simulink library "speedgoatlib"  (Simulink 7.5)
settings: Solver=ode45  StartTime=0.0  StopTime=10.0  RelTol=1e-3
undefined symbols (not defined in the file): m_XR17D15x, mmodemcontrol, standard
libraries: speedgoatlib x176, xpclib x88, simulink x4
(part 2 of 4)

== system speedgoatlib/IO503 ==
  Send Receive : Subsystem  InitFcn=m_XR17D15x(3);  mask(sendreceive_IO503){group=Basic Setup, port=1, irqnum=5, slot=-1, transceiver1=RS232 (max 921.6kb/s), standard1=on, baud1=115200, bauddivisor1=1, sampling1=16x (standard), prescale1=off, parity1=None, ndata1=8, nstop1=1, rlevel1=1, hwmode1=none, swmode1=none, xonchar1=17, xoffchar1=19, rs485auto1=off, rs485delay1=0, xmtfifosize1=1024, xmtdatatype1=8 bit uint null terminated, rcvfifosize1=1024, transceiver2=RS232 (max 921.6kb/s), standard2=on, baud2=115200, bauddivisor2=1, sampling2=16x (standard), prescale2=off, parity2=None, ndata2=8, nstop2=1, rlevel2=1, hwmode2=none, swmode2=none, xonchar2=17, xoffchar2=19, rs485auto2=off, rs485delay2=0, xmtfifosize2=1024, xmtdatatype2=8 bit uint null terminated, rcvfifosize2=1024, transceiver3=RS232 (max 921.6kb/s), standard3=on, baud3=115200, bauddivisor3=1, sampling3=16x (standard), prescale3=off, parity3=None, ndata3=8, nstop3=1, rlevel3=half full (32), hwmode3=none, swmode3=none, xonchar3=17, xoffchar3=19, rs485auto3=off, rs485delay3=0, xmtfifosize3=1024, xmtdatatype3=8 bit uint null terminated, rcvfifosize3=1024, transceiver4=RS232 (max 921.6kb/s), standard4=on, baud4=115200, bauddivisor4=1, sampling4=16x (standard), prescale4=off, parity4=None, ndata4=8, nstop4=1, rlevel4=half full (32), hwmode4=none, swmode4=none, xonchar4=17, xoffchar4=19, rs485auto4=off, rs485delay4=0, xmtfifosize4=1024, xmtdatatype4=8 bit uint null terminated, rcvfifosize4=1024}
      mask prompts: group "Parameter group:"; port "Port to modify:"; irqnum "IRQ number:"; slot "PCI slot (-1: autosearch):"; transceiver1 "Transceiver setup:"; standard1 "Use standard baud rates (16x, no prescaling)"; baud1 "Standard baud rate:"; bauddivisor1 "Baud rate divisor (non-standard baud rates):"; sampling1 "Sampling rate (non-standard baud rates):"; prescale1 "Prescale by 4 (non-standard baud rates)"; parity1 "Parity:"; ndata1 "Data bits:"; nstop1 "Stop bits:"; rlevel1 "Receive FIFO interrupt level:"; hwmode1 "Hardware handshake:"; swmode1 "Software handshake:"; xonchar1 "XON character:"; xoffchar1 "XOFF character:"; rs485auto1 "RS485 auto turnaround:"; rs485delay1 "RS485 turnaround delay [0,15]"; xmtfifosize1 "Transmit software FIFO size:"; xmtdatatype1 "Transmit FIFO data type:"; rcvfifosize1 "Receive software FIFO size:"; transceiver2 "Transceiver setup:"; standard2 "Use standard baud rates (16x, no prescaling)"; baud2 "Standard baud rate:"; bauddivisor2 "Baud rate divisor (non-standard baud rates):"; sampling2 "Sampling rate (non-standard baud rates):"; prescale2 "Prescale by 4 (non-standard baud rates)"; parity2 "Parity:"; ndata2 "Data bits:"; nstop2 "Stop bits:"; rlevel2 "Receive FIFO interrupt level:"; hwmode2 "Hardware handshake:"; swmode2 "Software handshake:"; xonchar2 "XON character:"; xoffchar2 "XOFF character:"; rs485auto2 "RS485 auto turnaround:"; rs485delay2 "RS485 turnaround delay [0,15]"; xmtfifosize2 "Transmit software FIFO size:"; xmtdatatype2 "Transmit FIFO data type:"; rcvfifosize2 "Receive software FIFO size:"; transceiver3 "Transceiver setup:"; standard3 "Use standard baud rates (16x, no prescaling)"; baud3 "Standard baud rate:"; bauddivisor3 "Baud rate divisor (non-standard baud rates):"; sampling3 "Sampling rate (non-standard baud rates):"; prescale3 "Prescale by 4 (non-standard baud rates)"; parity3 "Parity:"; ndata3 "Data bits:"; nstop3 "Stop bits:"; rlevel3 "Receive FIFO interrupt level:"; hwmode3 "Hardware handshake:"; swmode3 "Software handshake:"; xonchar3 "XON character:"; xoffchar3 "XOFF character:"; rs485auto3 "RS485 auto turnaround:"; rs485delay3 "RS485 turnaround delay [0,15]"; xmtfifosize3 "Transmit software FIFO size:"; xmtdatatype3 "Transmit FIFO data type:"; rcvfifosize3 "Receive software FIFO size:"; transceiver4 "Transceiver setup:"; standard4 "Use standard baud rates (16x, no prescaling)"; baud4 "Standard baud rate:"; bauddivisor4 "Baud rate divisor (non-standard baud rates):"; sampling4 "Sampling rate (non-standard baud rates):"; prescale4 "Prescale by 4 (non-standard baud rates)"; parity4 "Parity:"; ndata4 "Data bits:"; nstop4 "Stop bits:"; rlevel4 "Receive FIFO interrupt level:"; hwmode4 "Hardware handshake:"; swmode4 "Software handshake:"; xonchar4 "XON character:"; xoffchar4 "XOFF character:"; rs485auto4 "RS485 auto turnaround:"; rs485delay4 "RS485 turnaround delay [0,15]"; xmtfifosize4 "Transmit software FIFO size:"; xmtdatatype4 "Transmit FIFO data type:"; rcvfifosize4 "Receive software FIFO size:"
      mask help:
      | Speedgoat driver block
      | IO503 - Send Receive
      mask init:
      | brdslot = slot;
      | m_tews_XR17D15x(1, 4);
      mask Help: web(fullfile(speedgoatroot,'sg_help','serial','dialog_fields_send_rec_io503.htm'),'-helpbrowser');
      mask StyleString: popup(Board Setup|Basic Setup|FIFO Setup),popup(1|2|3|4),edit,edit,popup(RS232 (max 921.6kb/s)|RS422|RS422 multidrop|RS485 full-duplex|RS485 half-duplex),checkbox,popup(2764800|1382400|921600|460800|230400|115200|57600|38400|19200|9600|4800|2400|1200|600|400),edit,popup(8x|16x (standard)),checkbox,popup(None|Even|Odd|Mark|Space),popup(5|6|7|8),popup(1|2),popup(1|quarter full (16)|half full (32)|almost full (56)),popup(RTS/CTS|none),popup(XON/XOFF|none),edit,edit,checkbox,edit,edit,popup(count+32 bit int|count+32 bit uint|count+16 bit int|count+16 bit uint|8 bit int null terminated|8 bit uint null terminated),edit,popup(RS232 (max 921.6kb/s)|RS422|RS422 multidrop|RS485 full-duplex|RS485 half-duplex),checkbox,popup(2764800|1382400|921600|460800|230400|115200|57600|38400|19200|9600|4800|2400|1200|600|400),edit,popup(8x|16x (standard)),checkbox,popup(None|Even|Odd|Mark|Space),popup(5|6|7|8),popup(1|2),popup(1|quarter full (16)|half full (32)|almost full (56)),popup(RTS/CTS|none),popup(XON/XOFF|none),edit,edit,checkbox,edit,edit,popup(count+32 bit int|count+32 bit uint|count+16 bit int|count+16 bit uint|8 bit int null terminated|8 bit uint null terminated),edit,popup(RS232 (max 921.6kb/s)|RS422|RS422 multidrop|RS485 full-duplex|RS485 half-duplex),checkbox,popup(2764800|1382400|921600|460800|230400|115200|57600|38400|19200|9600|4800|2400|1200|600|400),edit,popup(8x|16x (standard)),checkbox,popup(None|Even|Odd|Mark|Space),popup(5|6|7|8),popup(1|2),popup(1|quarter full (16)|half full (32)|almost full (56)),popup(RTS/CTS|none),popup(XON/XOFF|none),edit,edit,checkbox,edit,edit,popup(count+32 bit int|count+32 bit uint|count+16 bit int|count+16 bit uint|8 bit int null terminated|8 bit uint null terminated),edit,popup(RS232 (max 921.6kb/s)|RS422|RS422 multidrop|RS485 full-duplex|RS485 half-duplex),checkbox,popup(2764800|1382400|921600|460800|230400|115200|57600|38400|19200|9600|4800|2400|1200|600|400),edit,popup(8x|16x (standard)),checkbox,popup(None|Even|Odd|Mark|Space),popup(5|6|7|8),popup(1|2),popup(1|quarter full (16)|half full (32)|almost full (56)),popup(RTS/CTS|none),popup(XON/XOFF|none),edit,edit,checkbox,edit,edit,popup(count+32 bit int|count+32 bit uint|count+16 bit int|count+16 bit uint|8 bit int null terminated|8 bit uint null terminated),edit
      mask CallbackString: m_tews_XR17D15x(2, 4);|m_tews_XR17D15x(2, 4);||||||||||||||||||||||||||||||||||||||||||||||||||||||||||||||||||||||||||||||
      mask Display:
      | disp('Speedgoat\nIO503\nRS232/422/485\nSend\nReceive');
      | port_label( 'input', 1, 'XMT1' );
      | port_label( 'input', 2, 'XMT2' );
      | port_label( 'input', 3, 'XMT3' );
      | port_label( 'input', 4, 'XMT4' );
      | 
      | port_label( 'output', 1, 'FIFO1' );
      | port_label( 'output', 2, 'FIFO2' );
      | port_label( 'output', 3, 'FIFO3' );
      | port_label( 'output', 4, 'FIFO4' );
  Speedgoat IO503 Internal blocks : Subsystem

== system speedgoatlib/IO504 ==
  Send Receive : Subsystem  InitFcn=m_XR17D15x(3);  mask(sendreceive_IO504){group=Basic Setup, port=1, irqnum=5, slot=-1, transceiver1=RS232 (max 921.6kb/s), standard1=on, baud1=115200, bauddivisor1=1, sampling1=16x (standard), prescale1=off, parity1=None, ndata1=8, nstop1=1, rlevel1=1, hwmode1=none, swmode1=none, xonchar1=17, xoffchar1=19, rs485auto1=off, rs485delay1=0, xmtfifosize1=1024, xmtdatatype1=8 bit uint null terminated, rcvfifosize1=1024, transceiver2=RS232 (max 921.6kb/s), standard2=on, baud2=115200, bauddivisor2=1, sampling2=16x (standard), prescale2=off, parity2=None, ndata2=8, nstop2=1, rlevel2=1, hwmode2=none, swmode2=none, xonchar2=17, xoffchar2=19, rs485auto2=off, rs485delay2=0, xmtfifosize2=1024, xmtdatatype2=8 bit uint null terminated, rcvfifosize2=1024, transceiver3=RS232 (max 921.6kb/s), standard3=on, baud3=115200, bauddivisor3=1, sampling3=16x (standard), prescale3=off, parity3=None, ndata3=8, nstop3=1, rlevel3=half full (32), hwmode3=none, swmode3=none, xonchar3=17, xoffchar3=19, rs485auto3=off, rs485delay3=0, xmtfifosize3=1024, xmtdatatype3=8 bit uint null terminated, rcvfifosize3=1024, transceiver4=RS232 (max 921.6kb/s), standard4=on, baud4=115200, bauddivisor4=1, sampling4=16x (standard), prescale4=off, parity4=None, ndata4=8, nstop4=1, rlevel4=half full (32), hwmode4=none, swmode4=none, xonchar4=17, xoffchar4=19, rs485auto4=off, rs485delay4=0, xmtfifosize4=1024, xmtdatatype4=8 bit uint null terminated, rcvfifosize4=1024, transceiver5=RS232 (max 921.6kb/s), standard5=on, baud5=115200, bauddivisor5=1, sampling5=16x (standard), prescale5=off, parity5=None, ndata5=8, nstop5=1, rlevel5=1, hwmode5=none, swmode5=none, xonchar5=17, xoffchar5=19, rs485auto5=off, rs485delay5=0, xmtfifosize5=1024, xmtdatatype5=8 bit uint null terminated, rcvfifosize5=1024, transceiver6=RS232 (max 921.6kb/s), standard6=on, baud6=115200, bauddivisor6=1, sampling6=16x (standard), prescale6=off, parity6=None, ndata6=8, nstop6=1, rlevel6=1, hwmode6=none, swmode6=none, xonchar6=17, xoffchar6=19, rs485auto6=off, rs485delay6=0, xmtfifosize6=1024, xmtdatatype6=8 bit uint null terminated, rcvfifosize6=1024, transceiver7=RS232 (max 921.6kb/s), standard7=on, baud7=115200, bauddivisor7=1, sampling7=16x (standard), prescale7=off, parity7=None, ndata7=8, nstop7=1, rlevel7=1, hwmode7=none, swmode7=none, xonchar7=17, xoffchar7=19, rs485auto7=off, rs485delay7=0, xmtfifosize7=1024, xmtdatatype7=8 bit uint null terminated, rcvfifosize7=1024, transceiver8=RS232 (max 921.6kb/s), standard8=on, baud8=115200, bauddivisor8=1, sampling8=16x (standard), prescale8=off, parity8=None, ndata8=8, nstop8=1, rlevel8=1, hwmode8=none, swmode8=none, xonchar8=17, xoffchar8=19, rs485auto8=off, rs485delay8=0, xmtfifosize8=1024, xmtdatatype8=8 bit uint null terminated, rcvfifosize8=1024}
      mask prompts: group "Parameter group:"; port "Port to modify:"; irqnum "IRQ number:"; slot "PCI slot (-1: autosearch):"; transceiver1 "Transceiver setup:"; standard1 "Use standard baud rates (16x, no prescaling)"; baud1 "Standard baud rate:"; bauddivisor1 "Baud rate divisor (non-standard baud rates):"; sampling1 "Sampling rate (non-standard baud rates):"; prescale1 "Prescale by 4 (non-standard baud rates)"; parity1 "Parity:"; ndata1 "Data bits:"; nstop1 "Stop bits:"; rlevel1 "Receive FIFO interrupt level:"; hwmode1 "Hardware handshake:"; swmode1 "Software handshake:"; xonchar1 "XON character:"; xoffchar1 "XOFF character:"; rs485auto1 "RS485 auto turnaround:"; rs485delay1 "RS485 turnaround delay [0,15]"; xmtfifosize1 "Transmit software FIFO size:"; xmtdatatype1 "Transmit FIFO data type:"; rcvfifosize1 "Receive software FIFO size:"; transceiver2 "Transceiver setup:"; standard2 "Use standard baud rates (16x, no prescaling)"; baud2 "Standard baud rate:"; bauddivisor2 "Baud rate divisor (non-standard baud rates):"; sampling2 "Sampling rate (non-standard baud rates):"; prescale2 "Prescale by 4 (non-standard baud rates)"; parity2 "Parity:"; ndata2 "Data bits:"; nstop2 "Stop bits:"; rlevel2 "Receive FIFO interrupt level:"; hwmode2 "Hardware handshake:"; swmode2 "Software handshake:"; xonchar2 "XON character:"; xoffchar2 "XOFF character:"; rs485auto2 "RS485 auto turnaround:"; rs485delay2 "RS485 turnaround delay [0,15]"; xmtfifosize2 "Transmit software FIFO size:"; xmtdatatype2 "Transmit FIFO data type:"; rcvfifosize2 "Receive software FIFO size:"; transceiver3 "Transceiver setup:"; standard3 "Use standard baud rates (16x, no prescaling)"; baud3 "Standard baud rate:"; bauddivisor3 "Baud rate divisor (non-standard baud rates):"; sampling3 "Sampling rate (non-standard baud rates):"; prescale3 "Prescale by 4 (non-standard baud rates)"; parity3 "Parity:"; ndata3 "Data bits:"; nstop3 "Stop bits:"; rlevel3 "Receive FIFO interrupt level:"; hwmode3 "Hardware handshake:"; swmode3 "Software handshake:"; xonchar3 "XON character:"; xoffchar3 "XOFF character:"; rs485auto3 "RS485 auto turnaround:"; rs485delay3 "RS485 turnaround delay [0,15]"; xmtfifosize3 "Transmit software FIFO size:"; xmtdatatype3 "Transmit FIFO data type:"; rcvfifosize3 "Receive software FIFO size:"; transceiver4 "Transceiver setup:"; standard4 "Use standard baud rates (16x, no prescaling)"; baud4 "Standard baud rate:"; bauddivisor4 "Baud rate divisor (non-standard baud rates):"; sampling4 "Sampling rate (non-standard baud rates):"; prescale4 "Prescale by 4 (non-standard baud rates)"; parity4 "Parity:"; ndata4 "Data bits:"; nstop4 "Stop bits:"; rlevel4 "Receive FIFO interrupt level:"; hwmode4 "Hardware handshake:"; swmode4 "Software handshake:"; xonchar4 "XON character:"; xoffchar4 "XOFF character:"; rs485auto4 "RS485 auto turnaround:"; rs485delay4 "RS485 turnaround delay [0,15]"; xmtfifosize4 "Transmit software FIFO size:"; xmtdatatype4 "Transmit FIFO data type:"; rcvfifosize4 "Receive software FIFO size:"; transceiver5 "Transceiver setup:"; standard5 "Use standard baud rates (16x, no prescaling)"; baud5 "Standard baud rate:"; bauddivisor5 "Baud rate divisor (non-standard baud rates):"; sampling5 "Sampling rate (non-standard baud rates):"; prescale5 "Prescale by 4 (non-standard baud rates)"; parity5 "Parity:"; ndata5 "Data bits:"; nstop5 "Stop bits:"; rlevel5 "Receive FIFO interrupt level:"; hwmode5 "Hardware handshake:"; swmode5 "Software handshake:"; xonchar5 "XON character:"; xoffchar5 "XOFF character:"; rs485auto5 "RS485 auto turnaround:"; rs485delay5 "RS485 turnaround delay [0,15]"; xmtfifosize5 "Transmit software FIFO size:"; xmtdatatype5 "Transmit FIFO data type:"; rcvfifosize5 "Receive software FIFO size:"; transceiver6 "Transceiver setup:"; standard6 "Use standard baud rates (16x, no prescaling)"; baud6 "Standard baud rate:"; bauddivisor6 "Baud rate divisor (non-standard baud rates):"; sampling6 "Sampling rate (non-standard baud rates):"; prescale6 "Prescale by 4 (non-standard baud rates)"; parity6 "Parity:"; ndata6 "Data bits:"; nstop6 "Stop bits:"; rlevel6 "Receive FIFO interrupt level:"; hwmode6 "Hardware handshake:"; swmode6 "Software handshake:"; xonchar6 "XON character:"; xoffchar6 "XOFF character:"; rs485auto6 "RS485 auto turnaround:"; rs485delay6 "RS485 turnaround delay [0,15]"; xmtfifosize6 "Transmit software FIFO size:"; xmtdatatype6 "Transmit FIFO data type:"; rcvfifosize6 "Receive software FIFO size:"; transceiver7 "Transceiver setup:"; standard7 "Use standard baud rates (16x, no prescaling)"; baud7 "Standard baud rate:"; bauddivisor7 "Baud rate divisor (non-standard baud rates):"; sampling7 "Sampling rate (non-standard baud rates):"; prescale7 "Prescale by 4 (non-standard baud rates)"; parity7 "Parity:"; ndata7 "Data bits:"; nstop7 "Stop bits:"; rlevel7 "Receive FIFO interrupt level:"; hwmode7 "Hardware handshake:"; swmode7 "Software handshake:"; xonchar7 "XON character:"; xoffchar7 "XOFF character:"; rs485auto7 "RS485 auto turnaround:"; rs485delay7 "RS485 turnaround delay [0,15]"; xmtfifosize7 "Transmit software FIFO size:"; xmtdatatype7 "Transmit FIFO data type:"; rcvfifosize7 "Receive software FIFO size:"; transceiver8 "Transceiver setup:"; standard8 "Use standard baud rates (16x, no prescaling)"; baud8 "Standard baud rate:"; bauddivisor8 "Baud rate divisor (non-standard baud rates):"; sampling8 "Sampling rate (non-standard baud rates):"; prescale8 "Prescale by 4 (non-standard baud rates)"; parity8 "Parity:"; ndata8 "Data bits:"; nstop8 "Stop bits:"; rlevel8 "Receive FIFO interrupt level:"; hwmode8 "Hardware handshake:"; swmode8 "Software handshake:"; xonchar8 "XON character:"; xoffchar8 "XOFF character:"; rs485auto8 "RS485 auto turnaround:"; rs485delay8 "RS485 turnaround delay [0,15]"; xmtfifosize8 "Transmit software FIFO size:"; xmtdatatype8 "Transmit FIFO data type:"; rcvfifosize8 "Receive software FIFO size:"
      mask help:
      | Speedgoat driver block
      | IO504 - Send Receive
      mask init:
      | brdslot = slot;
      | m_tews_XR17D15x(1, 8);
      mask Help: web(fullfile(speedgoatroot,'sg_help','serial','dialog_fields_send_rec_io503.htm'),'-helpbrowser');
      mask StyleString: popup(Board Setup|Basic Setup|FIFO Setup),popup(1|2|3|4|5|6|7|8),edit,edit,popup(RS232 (max 921.6kb/s)|RS422|RS422 multidrop|RS485 full-duplex|RS485 half-duplex),checkbox,popup(2764800|1382400|921600|460800|230400|115200|57600|38400|19200|9600|4800|2400|1200|600|400),edit,popup(8x|16x (standard)),checkbox,popup(None|Even|Odd|Mark|Space),popup(5|6|7|8),popup(1|2),popup(1|quarter full (16)|half full (32)|almost full (56)),popup(RTS/CTS|none),popup(XON/XOFF|none),edit,edit,checkbox,edit,edit,popup(count+32 bit int|count+32 bit uint|count+16 bit int|count+16 bit uint|8 bit int null terminated|8 bit uint null terminated),edit,popup(RS232 (max 921.6kb/s)|RS422|RS422 multidrop|RS485 full-duplex|RS485 half-duplex),checkbox,popup(2764800|1382400|921600|460800|230400|115200|57600|38400|19200|9600|4800|2400|1200|600|400),edit,popup(8x|16x (standard)),checkbox,popup(None|Even|Odd|Mark|Space),popup(5|6|7|8),popup(1|2),popup(1|quarter full (16)|half full (32)|almost full (56)),popup(RTS/CTS|none),popup(XON/XOFF|none),edit,edit,checkbox,edit,edit,popup(count+32 bit int|count+32 bit uint|count+16 bit int|count+16 bit uint|8 bit int null terminated|8 bit uint null terminated),edit,popup(RS232 (max 921.6kb/s)|RS422|RS422 multidrop|RS485 full-duplex|RS485 half-duplex),checkbox,popup(2764800|1382400|921600|460800|230400|115200|57600|38400|19200|9600|4800|2400|1200|600|400),edit,popup(8x|16x (standard)),checkbox,popup(None|Even|Odd|Mark|Space),popup(5|6|7|8),popup(1|2),popup(1|quarter full (16)|half full (32)|almost full (56)),popup(RTS/CTS|none),popup(XON/XOFF|none),edit,edit,checkbox,edit,edit,popup(count+32 bit int|count+32 bit uint|count+16 bit int|count+16 bit uint|8 bit int null terminated|8 bit uint null terminated),edit,popup(RS232 (max 921.6kb/s)|RS422|RS422 multidrop|RS485 full-duplex|RS485 half-duplex),checkbox,popup(2764800|1382400|921600|460800|230400|115200|57600|38400|19200|9600|4800|2400|1200|600|400),edit,popup(8x|16x (standard)),checkbox,popup(None|Even|Odd|Mark|Space),popup(5|6|7|8),popup(1|2),popup(1|quarter full (16)|half full (32)|almost full (56)),popup(RTS/CTS|none),popup(XON/XOFF|none),edit,edit,checkbox,edit,edit,popup(count+32 bit int|count+32 bit uint|count+16 bit int|count+16 bit uint|8 bit int null terminated|8 bit uint null terminated),edit,popup(RS232 (max 921.6kb/s)|RS422|RS422 multidrop|RS485 full-duplex|RS485 half-duplex),checkbox,popup(2764800|1382400|921600|460800|230400|115200|57600|38400|19200|9600|4800|2400|1200|600|400),edit,popup(8x|16x (standard)),checkbox,popup(None|Even|Odd|Mark|Space),popup(5|6|7|8),popup(1|2),popup(1|quarter full (16)|half full (32)|almost full (56)),popup(RTS/CTS|none),popup(XON/XOFF|none),edit,edit,checkbox,edit,edit,popup(count+32 bit int|count+32 bit uint|count+16 bit int|count+16 bit uint|8 bit int null terminated|8 bit uint null terminated),edit,popup(RS232 (max 921.6kb/s)|RS422|RS422 multidrop|RS485 full-duplex|RS485 half-duplex),checkbox,popup(2764800|1382400|921600|460800|230400|115200|57600|38400|19200|9600|4800|2400|1200|600|400),edit,popup(8x|16x (standard)),checkbox,popup(None|Even|Odd|Mark|Space),popup(5|6|7|8),popup(1|2),popup(1|quarter full (16)|half full (32)|almost full (56)),popup(RTS/CTS|none),popup(XON/XOFF|none),edit,edit,checkbox,edit,edit,popup(count+32 bit int|count+32 bit uint|count+16 bit int|count+16 bit uint|8 bit int null terminated|8 bit uint null terminated),edit,popup(RS232 (max 921.6kb/s)|RS422|RS422 multidrop|RS485 full-duplex|RS485 half-duplex),checkbox,popup(2764800|1382400|921600|460800|230400|115200|57600|38400|19200|9600|4800|2400|1200|600|400),edit,popup(8x|16x (standard)),checkbox,popup(None|Even|Odd|Mark|Space),popup(5|6|7|8),popup(1|2),popup(1|quarter full (16)|half full (32)|almost full (56)),popup(RTS/CTS|none),popup(XON/XOFF|none),edit,edit,checkbox,edit,edit,popup(count+32 bit int|count+32 bit uint|count+16 bit int|count+16 bit uint|8 bit int null terminated|8 bit uint null terminated),edit,popup(RS232 (max 921.6kb/s)|RS422|RS422 multidrop|RS485 full-duplex|RS485 half-duplex),checkbox,popup(2764800|1382400|921600|460800|230400|115200|57600|38400|19200|9600|4800|2400|1200|600|400),edit,popup(8x|16x (standard)),checkbox,popup(None|Even|Odd|Mark|Space),popup(5|6|7|8),popup(1|2),popup(1|quarter full (16)|half full (32)|almost full (56)),popup(RTS/CTS|none),popup(XON/XOFF|none),edit,edit,checkbox,edit,edit,popup(count+32 bit int|count+32 bit uint|count+16 bit int|count+16 bit uint|8 bit int null terminated|8 bit uint null terminated),edit
      mask CallbackString: m_tews_XR17D15x(2, 8);|m_tews_XR17D15x(2, 8);||||||||||||||||||||||||||||||||||||||||||||||||||||||||||||||||||||||||||||||||||||||||||||||||||||||||||||||||||||||||||||||||||||||||||||||||||||||||||
      mask Display:
      | disp('Speedgoat\nIO504\nRS232/422/485\nSend\nReceive');
      | port_label( 'input', 1, 'XMT1' );
      | port_label( 'input', 2, 'XMT2' );
      | port_label( 'input', 3, 'XMT3' );
      | port_label( 'input', 4, 'XMT4' );
      | port_label( 'input', 5, 'XMT5' );
      | port_label( 'input', 6, 'XMT6' );
      | port_label( 'input', 7, 'XMT7' );
      | port_label( 'input', 8, 'XMT8' );
      | 
      | port_label( 'output', 1, 'FIFO1' );
      | port_label( 'output', 2, 'FIFO2' );
      | port_label( 'output', 3, 'FIFO3' );
      | port_label( 'output', 4, 'FIFO4' );
      | port_label( 'output', 5, 'FIFO5' );
      | port_label( 'output', 6, 'FIFO6' );
      | port_label( 'output', 7, 'FIFO7' );
      | port_label( 'output', 8, 'FIFO8' );
  Speedgoat IO504 Internal blocks : Subsystem

== system speedgoatlib/IO511 ==

== system speedgoatlib/IO601 ==

== system speedgoatlib/IO642 ==

== system speedgoatlib/IO671 ==

== system speedgoatlib/IO681 ==

== system speedgoatlib/IO70X Fast Eth ==

== system speedgoatlib/IO71X Gigabit Eth ==

== system speedgoatlib/IO75x ==

== system speedgoatlib/IO901 IO902 ==

== system speedgoatlib/IO903 ==

== system speedgoatlib/IO907 ==

== system speedgoatlib/IO92x - IO971 ==

== system speedgoatlib/IO976 ==

== system speedgoatlib/Utilities ==

== system speedgoatlib/IO501/Acromag PMC520 Internal blocks ==
  Board Setup : S-Function  FunctionName=board_setup_XR17D15x  Parameters=slot, irqnum+4, 100, reffreq  EnableBusSupport=off  mask(board_setup_XR17D15x){reffreq=14745600, irqnum=5, slot=-1}
      mask prompts: reffreq "Reference Freq (standard = 14745600)   (6 Mhz <= F <= 50 Mhz)"; irqnum "IRQ Line Number"; slot "PCI slot: (-1 for autosearch)"
      mask help:
      | PMC520
      | Acromag
      | Board Setup
      mask Help: helpview(fullfile(docroot, 'mapfiles', 'xpc.map'), 'Commtech_422335_IntChk')
      mask StyleString: edit,popup(5|6|7|8|9|10|11|12|13|14|15),edit
      mask Display: disp('PMC520\nAcromag\nBoard Setup');
  "Enable TX " : S-Function  FunctionName=tx_int_enable_XR17D15x  Parameters=slot, port, 100  EnableBusSupport=off  mask(tx_int_enable_XR17D15x){port=1, slot=-1}
      mask prompts: slot "PCI slot: (-1 for autosearch)"
      mask help:
      | PMC520
      | Acromag
      | Enable TX Interrupt
      mask Help: helpview(fullfile(docroot, 'mapfiles', 'xpc.map'), 'FC422335_Enable_Int')
      mask StyleString: popup(1|2|3|4|5|6|7|8),edit
      mask Display:
      | disp('PMC520\nAcromag\nEnable TX int');
      | port_label('input', 1, 'E');
  Int Source Filter : S-Function  FunctionName=int_source_filter_XR17D15x  Parameters=port, 100, value  EnableBusSupport=off  mask(int_source_filter_XR17D15x){port=1, value=Receive data}
      mask prompts: value "Filter value:"
      mask help:
      | PMC520
      | Acromag
      | Interrupt Source Filter
      mask Help: helpview(fullfile(docroot, 'mapfiles', 'xpc.map'), 'FC422335_Filter_Ints')
      mask StyleString: popup(1|2|3|4|5|6|7|8),popup(Receive data|Transmitter empty|Modem status change)
      mask Display:
      | disp('PMC520\nAcromag\nInt Source Filter');
      | port_label('input', 1, 'S' );
      | port_label('output', 1, 'E' );
  Read HW FIFO : S-Function  FunctionName=read_hw_fifo_XR17D15x  Parameters=slot, port, 100, flush  EnableBusSupport=off  mask(read_hw_fifo_XR17D15x){port=1, flush=on, slot=-1}
      mask prompts: flush "Flush HW FIFO on startup"; slot "PCI slot: (-1 for autosearch)"
      mask help:
      | PMC520
      | Acromag
      | Read Hardware FIFO
      mask Help: helpview(fullfile(docroot, 'mapfiles', 'xpc.map'), 'FC422335_Read_HW')
      mask StyleString: popup(1|2|3|4|5|6|7|8),checkbox,edit
      mask Display:
      | disp('PMC520\nAcromag\nRead HW FIFO');
      | port_label('input', 1, 'E');
      | port_label('output', 1, 'D');
  Read Int Status : S-Function  FunctionName=read_int_status_XR17D15x  Parameters=slot, 100  EnableBusSupport=off  mask(read_int_status_XR17D15x){slot=-1}
      mask prompts: slot "PCI slot: (-1 for autosearch)"
      mask help:
      | PMC520
      | Acromag
      | Read Interrupt Status
      mask Help: helpview(fullfile(docroot, 'mapfiles', 'xpc.map'), 'Commtech_422335_Interrupt_Query')
      mask Display:
      | disp('PMC520\nAcromag\nRead Int Status');
      | port_label('output', 1, 'S' );
  "Setup " : S-Function  FunctionName=setup_XR17D15x  Parameters=slot, 100, port, standard, baudrate, bauddivisor, mode8x, prescale, width, nstop, parity, rlevel, ctsmode, xonoff, xon, xoff, rs485mode, rs485delay  EnableBusSupport=off  mask(setup_XR17D15x){port=1, standard=on, baudrate=115200, bauddivisor=1, mode8x=16x (standard), prescale=off, width=8, nstop=1, parity=None, rlevel=1, ctsmode=none, xonoff=none, xon=17, xoff=19, rs485mode=off, rs485delay=0, slot=-1}
      mask prompts: standard "Use standard reference and rates"; baudrate "Baud rate (using standard reference):"; bauddivisor "Baud Divisor (1 to 65535, custom rate):"; mode8x "Sampling rate:"; prescale "Prescale (Divide reference by 4)"; width "Number of data bits:"; nstop "Number of stop bits:"; rlevel "Receive trigger level:"; ctsmode "Hardware handshake:"; xonoff "Software handshake:"; xon "XON character:"; xoff "XOFF character:"; rs485mode "RS485 auto turnaround"; rs485delay "RS485 turnaround delay:"; slot "PCI slot: (-1 for autosearch)"
      mask help:
      | PMC520
      | Acromag
      | Setup
      mask Help: helpview(fullfile(docroot, 'mapfiles', 'xpc.map'), 'FC422335_Setup')
      mask StyleString: edit,checkbox,popup(921600|460800|230400|115200|57600|38400|19200|9600|4800|2400|1200|600|300|110),edit,popup(8x|16x (standard)),checkbox,popup(5|6|7|8),popup(1|2),popup(None|Even|Odd|Mark|Space),popup(1|quarter full (16)|half full (32)|almost full (56)),popup(RTS/CTS|DTR/DSR|none),popup(XON/XOFF|none),edit,edit,checkbox,edit,edit
      mask Display: disp('PMC520\nAcromag\nSetup');
  Write HW FIFO : S-Function  FunctionName=write_hw_fifo_XR17D15x  Parameters=slot, port, 100  EnableBusSupport=off  mask(write_hw_fifo_XR17D15x){port=1, slot=-1}
      mask prompts: slot "PCI slot: (-1 for autosearch)"
      mask help:
      | PMC520
      | Acromag
      | Write Hardware FIFO
      mask Help: helpview(fullfile(docroot, 'mapfiles', 'xpc.map'), 'FC422335_Write_HW')
      mask StyleString: popup(1|2|3|4|5|6|7|8),edit
      mask Display:
      | disp('PMC520\nAcromag\nWrite HW FIFO');
      | port_label('input', 1, 'D');
      | port_label('input', 2, 'E');

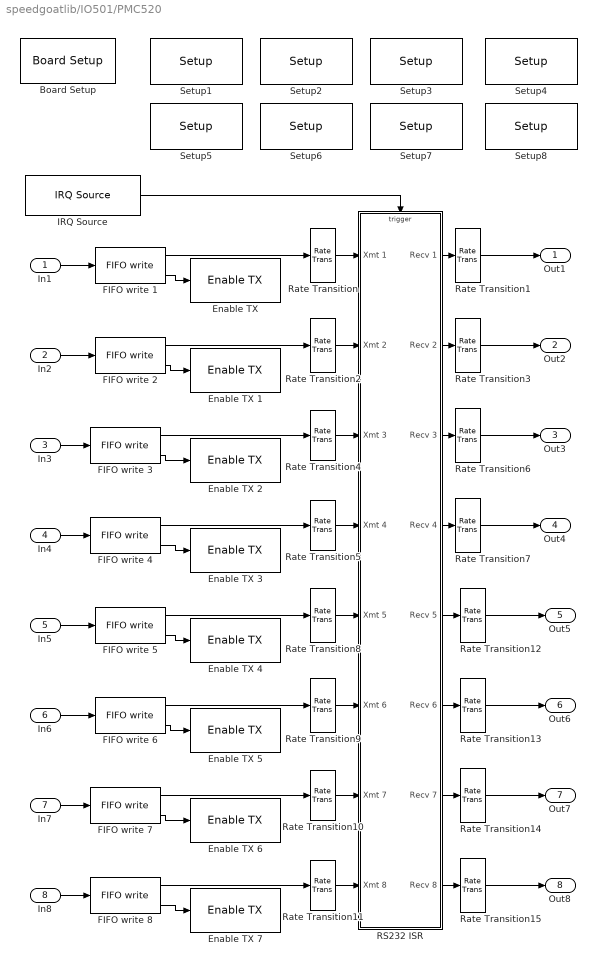
== system speedgoatlib/IO501/PMC520 ==
  In1 : Inport
  In2 : Inport  Port=2
  In3 : Inport  Port=3
  In4 : Inport  Port=4
  In5 : Inport  Port=5
  In6 : Inport  Port=6
  In7 : Inport  Port=7
  In8 : Inport  Port=8
  Board Setup : speedgoatlib/IO501/Acromag PMC520 Internal blocks/Board Setup  reffreq=14745600  irqnum=5  slot=brdslot
  "Enable TX " : speedgoatlib/IO501/Acromag PMC520 Internal blocks/Enable TX   port=1  slot=brdslot
  Enable TX 1 : speedgoatlib/IO501/Acromag PMC520 Internal blocks/Enable TX   port=2  slot=brdslot
  Enable TX 2 : speedgoatlib/IO501/Acromag PMC520 Internal blocks/Enable TX   port=3  slot=brdslot
  Enable TX 3 : speedgoatlib/IO501/Acromag PMC520 Internal blocks/Enable TX   port=4  slot=brdslot
  Enable TX 4 : speedgoatlib/IO501/Acromag PMC520 Internal blocks/Enable TX   port=5  slot=brdslot
  Enable TX 5 : speedgoatlib/IO501/Acromag PMC520 Internal blocks/Enable TX   port=6  slot=brdslot
  Enable TX 6 : speedgoatlib/IO501/Acromag PMC520 Internal blocks/Enable TX   port=7  slot=brdslot
  Enable TX 7 : speedgoatlib/IO501/Acromag PMC520 Internal blocks/Enable TX   port=8  slot=brdslot
  FIFO write 1 : xpclib/RS232/FIFO write   size=1024  inputtype=8 bit uint null terminated  present=on  sampletime=-1  id=XMT channel 1, IRQ 5
  FIFO write 2 : xpclib/RS232/FIFO write   size=1024  inputtype=8 bit uint null terminated  present=on  sampletime=-1  id=XMT channel 2, IRQ 5
  FIFO write 3 : xpclib/RS232/FIFO write   size=1024  inputtype=8 bit uint null terminated  present=on  sampletime=-1  id=XMT channel 3, IRQ 5
  FIFO write 4 : xpclib/RS232/FIFO write   size=1024  inputtype=8 bit uint null terminated  present=on  sampletime=-1  id=XMT channel 4, IRQ 5
  FIFO write 5 : xpclib/RS232/FIFO write   size=1024  inputtype=8 bit uint null terminated  present=on  sampletime=-1  id=XMT channel 5, IRQ 5
  FIFO write 6 : xpclib/RS232/FIFO write   size=1024  inputtype=8 bit uint null terminated  present=on  sampletime=-1  id=XMT channel 6, IRQ 5
  FIFO write 7 : xpclib/RS232/FIFO write   size=1024  inputtype=8 bit uint null terminated  present=on  sampletime=-1  id=XMT channel 7, IRQ 5
  FIFO write 8 : xpclib/RS232/FIFO write   size=1024  inputtype=8 bit uint null terminated  present=on  sampletime=-1  id=XMT channel 8, IRQ 5
  IRQ Source : xpclib/Asynchronous Event/IRQ Source  irqNo=5  preempt=off  b_type=None/Other  slot=brdslot
  RS232 ISR : Subsystem  TreatAsAtomicUnit=on  mask(RS232 ISR){slot=brdslot}
      mask help:
      | PMC520
      | Acromag
      | Interrupt Service Routine
      mask init:
      | subslot = slot;
      mask Display:
      | disp('PMC521\nAcromag\nISR');
      | port_label('input', 1, 'XMT1');
      | port_label('input', 2, 'XMT2');
      | port_label('input', 3, 'XMT3');
      | port_label('input', 4, 'XMT4');
      | port_label('input', 5, 'XMT5');
      | port_label('input', 6, 'XMT6');
      | port_label('input', 7, 'XMT7');
      | port_label('input', 8, 'XMT8');
      | port_label('output', 1, 'RCV1');
      | port_label('output', 2, 'RCV2');
      | port_label('output', 3, 'RCV3');
      | port_label('output', 4, 'RCV4');
      | port_label('output', 5, 'RCV5');
      | port_label('output', 6, 'RCV6');
      | port_label('output', 7, 'RCV7');
      | port_label('output', 8, 'RCV8');
  Rate Transition{,2,4..5,8..11} (8 alike) : RateTransition  Integrity=off  Deterministic=off
  Rate Transition{1,3,6..7,12..15} (8 alike) : RateTransition  Integrity=off  Deterministic=off  OutPortSampleTime=0
  Setup1 : speedgoatlib/IO501/Acromag PMC520 Internal blocks/Setup   port=1  standard=on  baudrate=115200  bauddivisor=1  mode8x=16x (standard)  prescale=off  width=8  nstop=1  parity=None  rlevel=1  ctsmode=none  xonoff=none  xon=17  xoff=19  rs485mode=off  rs485delay=0  slot=brdslot
  Setup2 : speedgoatlib/IO501/Acromag PMC520 Internal blocks/Setup   port=2  standard=on  baudrate=115200  bauddivisor=1  mode8x=16x (standard)  prescale=off  width=8  nstop=1  parity=None  rlevel=1  ctsmode=none  xonoff=none  xon=17  xoff=19  rs485mode=off  rs485delay=0  slot=brdslot
  Setup3 : speedgoatlib/IO501/Acromag PMC520 Internal blocks/Setup   port=3  standard=on  baudrate=115200  bauddivisor=1  mode8x=16x (standard)  prescale=off  width=8  nstop=1  parity=None  rlevel=half full (32)  ctsmode=none  xonoff=none  xon=17  xoff=19  rs485mode=off  rs485delay=0  slot=brdslot
  Setup4 : speedgoatlib/IO501/Acromag PMC520 Internal blocks/Setup   port=4  standard=on  baudrate=115200  bauddivisor=1  mode8x=16x (standard)  prescale=off  width=8  nstop=1  parity=None  rlevel=half full (32)  ctsmode=none  xonoff=none  xon=17  xoff=19  rs485mode=off  rs485delay=0  slot=brdslot
  Setup5 : speedgoatlib/IO501/Acromag PMC520 Internal blocks/Setup   port=5  standard=on  baudrate=115200  bauddivisor=1  mode8x=16x (standard)  prescale=off  width=8  nstop=1  parity=None  rlevel=1  ctsmode=none  xonoff=none  xon=17  xoff=19  rs485mode=off  rs485delay=0  slot=brdslot
  Setup6 : speedgoatlib/IO501/Acromag PMC520 Internal blocks/Setup   port=6  standard=on  baudrate=115200  bauddivisor=1  mode8x=16x (standard)  prescale=off  width=8  nstop=1  parity=None  rlevel=1  ctsmode=none  xonoff=none  xon=17  xoff=19  rs485mode=off  rs485delay=0  slot=brdslot
  Setup7 : speedgoatlib/IO501/Acromag PMC520 Internal blocks/Setup   port=7  standard=on  baudrate=115200  bauddivisor=1  mode8x=16x (standard)  prescale=off  width=8  nstop=1  parity=None  rlevel=1  ctsmode=none  xonoff=none  xon=17  xoff=19  rs485mode=off  rs485delay=0  slot=brdslot
  Setup8 : speedgoatlib/IO501/Acromag PMC520 Internal blocks/Setup   port=8  standard=on  baudrate=115200  bauddivisor=1  mode8x=16x (standard)  prescale=off  width=8  nstop=1  parity=None  rlevel=1  ctsmode=none  xonoff=none  xon=17  xoff=19  rs485mode=off  rs485delay=0  slot=brdslot
  Out1 : Outport
  Out2 : Outport  Port=2
  Out3 : Outport  Port=3
  Out4 : Outport  Port=4
  Out5 : Outport  Port=5
  Out6 : Outport  Port=6
  Out7 : Outport  Port=7
  Out8 : Outport  Port=8
  wires:
  RS232 ISR/4(Recv 4) -> Rate Transition7/1
  RS232 ISR/3(Recv 3) -> Rate Transition6/1
  Rate Transition7/1 -> Out4/1
  Rate Transition6/1 -> Out3/1
  Rate Transition5/1 -> RS232 ISR/4(Xmt 4)
  Rate Transition4/1 -> RS232 ISR/3(Xmt 3)
  FIFO write 4/1 -> Rate Transition5/1
  In4/1 -> FIFO write 4/1
  FIFO write 4/2 -> Enable TX 3/1
  FIFO write 3/1 -> Rate Transition4/1
  In3/1 -> FIFO write 3/1
  FIFO write 3/2 -> Enable TX 2/1
  Rate Transition1/1 -> Out1/1
  Rate Transition3/1 -> Out2/1
  Rate Transition/1 -> RS232 ISR/1(Xmt 1)
  Rate Transition2/1 -> RS232 ISR/2(Xmt 2)
  FIFO write 1/2 -> "Enable TX "/1
  IRQ Source/1 -> RS232 ISR/Trigger
  RS232 ISR/1(Recv 1) -> Rate Transition1/1
  RS232 ISR/2(Recv 2) -> Rate Transition3/1
  FIFO write 1/1 -> Rate Transition/1
  In1/1 -> FIFO write 1/1
  FIFO write 2/1 -> Rate Transition2/1
  In2/1 -> FIFO write 2/1
  FIFO write 2/2 -> Enable TX 1/1
  Rate Transition11/1 -> RS232 ISR/8(Xmt 8)
  Rate Transition10/1 -> RS232 ISR/7(Xmt 7)
  FIFO write 8/1 -> Rate Transition11/1
  In8/1 -> FIFO write 8/1
  FIFO write 8/2 -> Enable TX 7/1
  FIFO write 7/1 -> Rate Transition10/1
  In7/1 -> FIFO write 7/1
  FIFO write 7/2 -> Enable TX 6/1
  Rate Transition8/1 -> RS232 ISR/5(Xmt 5)
  Rate Transition9/1 -> RS232 ISR/6(Xmt 6)
  FIFO write 5/2 -> Enable TX 4/1
  FIFO write 5/1 -> Rate Transition8/1
  In5/1 -> FIFO write 5/1
  FIFO write 6/1 -> Rate Transition9/1
  In6/1 -> FIFO write 6/1
  FIFO write 6/2 -> Enable TX 5/1
  Rate Transition15/1 -> Out8/1
  Rate Transition14/1 -> Out7/1
  Rate Transition12/1 -> Out5/1
  Rate Transition13/1 -> Out6/1
  RS232 ISR/5(Recv 5) -> Rate Transition12/1
  RS232 ISR/6(Recv 6) -> Rate Transition13/1
  RS232 ISR/7(Recv 7) -> Rate Transition14/1
  RS232 ISR/8(Recv 8) -> Rate Transition15/1

== system speedgoatlib/IO502/Acromag PMC521 Internal blocks ==
  Board Setup : S-Function  FunctionName=board_setup_XR17D15x  Parameters=slot, irqnum+4, 101, reffreq  EnableBusSupport=off  mask(board_setup_XR17D15x){reffreq=14745600, irqnum=5, slot=-1}
      mask prompts: reffreq "Reference Freq (standard = 14745600)   (6 Mhz <= F <= 50 Mhz)"; irqnum "IRQ Line Number"; slot "PCI slot: (-1 for autosearch)"
      mask help:
      | PMC521
      | Acromag
      | Board Setup
      mask Help: helpview(fullfile(docroot, 'mapfiles', 'xpc.map'), 'Commtech_422335_IntChk')
      mask StyleString: edit,popup(5|6|7|8|9|10|11|12|13|14|15),edit
      mask Display: disp('PMC521\nAcromag\nBoard Setup');
  Disable Transmitter 1 : S-Function  FunctionName=RxD_enable_PMC521_XR17D15x  Parameters=slot, port, 101  EnableBusSupport=off  mask(tx_int_enable_XR17D15x){port=1, slot=-1}
      mask prompts: slot "PCI slot: (-1 for autosearch)"
      mask help:
      | PMC521
      | Acromag
      | Enable TX Interrupt
      mask Help: helpview(fullfile(docroot, 'mapfiles', 'xpc.map'), 'FC422335_Enable_Int')
      mask StyleString: popup(1|2|3|4|5|6|7|8),edit
      mask Display:
      | disp('PMC521\nAcromag\nDisable Transmitter');
      | port_label('input', 1, 'E');
  "Enable TX " : S-Function  FunctionName=tx_int_enable_XR17D15x  Parameters=slot, port, 101  EnableBusSupport=off  mask(tx_int_enable_XR17D15x){port=1, slot=-1}
      mask prompts: slot "PCI slot: (-1 for autosearch)"
      mask help:
      | PMC521
      | Acromag
      | Enable TX Interrupt
      mask Help: helpview(fullfile(docroot, 'mapfiles', 'xpc.map'), 'FC422335_Enable_Int')
      mask StyleString: popup(1|2|3|4|5|6|7|8),edit
      mask Display:
      | disp('PMC521\nAcromag\nEnable TX int');
      | port_label('input', 1, 'E');
  Enhanced Write HW FIFO 1 : S-Function  FunctionName=write_hw_fifo_PMC521_XR17D15x  Parameters=slot, port, 101, halfduplex  EnableBusSupport=off  mask(write_hw_fifo_XR17D15x){port=1, halfduplex=on, slot=-1}
      mask prompts: halfduplex "Enable transmitter at entry"; slot "PCI slot: (-1 for autosearch)"
      mask help:
      | PMC521
      | Acromag
      | Write Hardware FIFO
      mask Help: helpview(fullfile(docroot, 'mapfiles', 'xpc.map'), 'FC422335_Write_HW')
      mask StyleString: popup(1|2|3|4|5|6|7|8),checkbox,edit
      mask Display:
      | disp('PMC521\nAcromag\nEnhanced Write HW FIFO');
      | port_label('input', 1, 'D');
      | port_label('input', 2, 'E');
  Int Source Filter : S-Function  FunctionName=int_source_filter_XR17D15x  Parameters=port, 101, value  EnableBusSupport=off  mask(int_source_filter_XR17D15x){port=1, value=Receive data}
      mask prompts: value "Filter value:"
      mask help:
      | PMC521
      | Acromag
      | Interrupt Source Filter
      mask Help: helpview(fullfile(docroot, 'mapfiles', 'xpc.map'), 'FC422335_Filter_Ints')
      mask StyleString: popup(1|2|3|4|5|6|7|8),popup(Receive data|Transmitter empty|Modem status change)
      mask Display:
      | disp('PMC521\nAcromag\nInt Source Filter');
      | port_label('input', 1, 'S' );
      | port_label('output', 1, 'E' );
  Read HW FIFO : S-Function  FunctionName=read_hw_fifo_XR17D15x  Parameters=slot, port, 101, flush  EnableBusSupport=off  mask(read_hw_fifo_XR17D15x){port=1, flush=on, slot=-1}
      mask prompts: flush "Flush HW FIFO on startup"; slot "PCI slot: (-1 for autosearch)"
      mask help:
      | PMC521
      | Acromag
      | Read Hardware FIFO
      mask Help: helpview(fullfile(docroot, 'mapfiles', 'xpc.map'), 'FC422335_Read_HW')
      mask StyleString: popup(1|2|3|4|5|6|7|8),checkbox,edit
      mask Display:
      | disp('PMC521\nAcromag\nRead HW FIFO');
      | port_label('input', 1, 'E');
      | port_label('output', 1, 'D');
  Read Int Status : S-Function  FunctionName=read_int_status_XR17D15x  Parameters=slot, 101  EnableBusSupport=off  mask(read_int_status_XR17D15x){slot=-1}
      mask prompts: slot "PCI slot: (-1 for autosearch)"
      mask help:
      | PMC521
      | Acromag
      | Read Interrupt Status
      mask Help: helpview(fullfile(docroot, 'mapfiles', 'xpc.map'), 'Commtech_422335_Interrupt_Query')
      mask Display:
      | disp('PMC521\nAcromag\nRead Int Status');
      | port_label('output', 1, 'S' );
  "Setup " : S-Function  FunctionName=setup_XR17D15x  Parameters=slot, 101, port, standard, baudrate, bauddivisor, mode8x, prescale, width, nstop, parity, rlevel, ctsmode, xonoff, xon, xoff, rs485mode, rs485delay  EnableBusSupport=off  mask(setup_XR17D15x){port=1, standard=on, baudrate=115200, bauddivisor=1, mode8x=16x (standard), prescale=off, width=8, nstop=1, parity=None, rlevel=1, ctsmode=none, xonoff=none, xon=17, xoff=19, rs485mode=off, rs485delay=0, slot=-1}
      mask prompts: standard "Use standard reference and rates"; baudrate "Baud rate (using standard reference):"; bauddivisor "Baud Divisor (1 to 65535, custom rate):"; mode8x "Sampling rate:"; prescale "Prescale (Divide reference by 4)"; width "Number of data bits:"; nstop "Number of stop bits:"; rlevel "Receive trigger level:"; ctsmode "Hardware handshake:"; xonoff "Software handshake:"; xon "XON character:"; xoff "XOFF character:"; rs485mode "RS485 auto turnaround"; rs485delay "RS485 turnaround delay:"; slot "PCI slot: (-1 for autosearch)"
      mask help:
      | PMC521
      | Acromag
      | Setup
      mask Help: helpview(fullfile(docroot, 'mapfiles', 'xpc.map'), 'FC422335_Setup')
      mask StyleString: edit,checkbox,popup(921600|460800|230400|115200|57600|38400|19200|9600|4800|2400|1200|600|300|110),edit,popup(8x|16x (standard)),checkbox,popup(5|6|7|8),popup(1|2),popup(None|Even|Odd|Mark|Space),popup(1|quarter full (16)|half full (32)|almost full (56)),popup(RTS/CTS|DTR/DSR|none),popup(XON/XOFF|none),edit,edit,checkbox,edit,edit
      mask Display: disp('PMC521\nAcromag\nSetup');
  Setup 2 : S-Function  FunctionName=setup_PMC521_XR17D15x  Parameters=slot, 101, port, standard, baudrate, bauddivisor, mode8x, prescale, width, nstop, parity, rlevel, ctsmode, xonoff, xon, xoff, rs485mode, rs485delay, recint, mcrrts  EnableBusSupport=off  mask(setup_XR17D15x){port=1, standard=on, baudrate=115200, bauddivisor=1, mode8x=16x (standard), prescale=off, width=8, nstop=1, parity=None, rlevel=1, ctsmode=none, xonoff=none, xon=17, xoff=19, rs485mode=off, rs485delay=0, recint=on, mcrrts=on, slot=-1}
      mask prompts: standard "Use standard reference and rates"; baudrate "Baud rate (using standard reference):"; bauddivisor "Baud Divisor (1 to 65535, custom rate):"; mode8x "Sampling rate:"; prescale "Prescale (Divide reference by 4)"; width "Number of data bits:"; nstop "Number of stop bits:"; rlevel "Receive trigger level:"; ctsmode "Hardware handshake:"; xonoff "Software handshake:"; xon "XON character:"; xoff "XOFF character:"; rs485mode "RS485 auto turnaround"; rs485delay "RS485 turnaround delay:"; recint "Enable receive FIFO interrupts"; mcrrts "Enable transmitter"; slot "PCI slot: (-1 for autosearch)"
      mask help:
      | PMC521
      | Acromag
      | Setup
      mask Help: helpview(fullfile(docroot, 'mapfiles', 'xpc.map'), 'FC422335_Setup')
      mask StyleString: edit,checkbox,popup(921600|460800|230400|115200|57600|38400|19200|9600|4800|2400|1200|600|300|110),edit,popup(8x|16x (standard)),checkbox,popup(5|6|7|8),popup(1|2),popup(None|Even|Odd|Mark|Space),popup(1|quarter full (16)|half full (32)|almost full (56)),popup(RTS/CTS|DTR/DSR|none),popup(XON/XOFF|none),edit,edit,checkbox,edit,checkbox,checkbox,edit
      mask Display: disp('PMC521\nAcromag\nEnhanced Setup');
  Write HW FIFO : S-Function  FunctionName=write_hw_fifo_XR17D15x  Parameters=slot, port, 101  EnableBusSupport=off  mask(write_hw_fifo_XR17D15x){port=1, slot=-1}
      mask prompts: slot "PCI slot: (-1 for autosearch)"
      mask help:
      | PMC521
      | Acromag
      | Write Hardware FIFO
      mask Help: helpview(fullfile(docroot, 'mapfiles', 'xpc.map'), 'FC422335_Write_HW')
      mask StyleString: popup(1|2|3|4|5|6|7|8),edit
      mask Display:
      | disp('PMC521\nAcromag\nWrite HW FIFO');
      | port_label('input', 1, 'D');
      | port_label('input', 2, 'E');
